simulink model "verify_Flow_Mixer_Thermostatic_mdl"  (R2016b)
settings: Solver=ode45  StartTime=0.0  StopTime=600  MaxStep=1  RelTol=1e-3  EnableMultiTasking=on
libraries: carnot x7, simulink x2
settings Model: DEBUGGLOBALLEVEL=NOLEVEL  DEBUGMAXTOTALWARNINGS=inf  DEBUGMAXCONSECUTIVEWARNINGS=inf  DEBUGWRITETOFILE=0  DEBUGFILENAME='error.txt'  Creator=drhf  LastModifiedBy=drhf
settings DataIOCC: SaveFormat=Array  SignalLoggingSaveFormat=ModelDataLogs
settings OptimizationCC: ExpressionDepthLimit=2147483647  LifeSpan=inf
settings DebuggingCC: UnderspecifiedInitializationDetection=Classic  MergeDetectMultiDrivingBlocksExec=none  SolverPrmCheckMsg=warning  FcnCallInpInsideContextMsg=warning  StateNameClashWarn=warning  SFUnexpectedBacktrackingDiag=warning  SFNoUnconditionalDefaultTransitionDiag=warning  SFExecutionAtInitializationDiag=none
settings HardwareCC: ProdBitPerPointer=32  ProdBitPerSizeT=32  ProdBitPerPtrDiffT=32  ProdLargestAtomicFloat=None  ProdIntDivRoundTo=Undefined  ProdEndianess=Unspecified  ProdWordSize=32  ProdHWDeviceType=32-bit Generic
settings ModelReferenceCC: PropagateSignalLabelsOutOfModel=off
settings GRTTargetCC: TargetLangStandard=C89/C90 (ANSI)  GeneratePreprocessorConditionals=Disable all  CombineOutputUpdateFcns=off  GRTInterface=on
settings ConfigComp: CovMetricSettings=dw  CovHtmlReporting=on  CovSaveCumulativeToWorkspaceVar=on  CovSaveSingleToWorkspaceVar=on  CovExternalEMLEnable=off

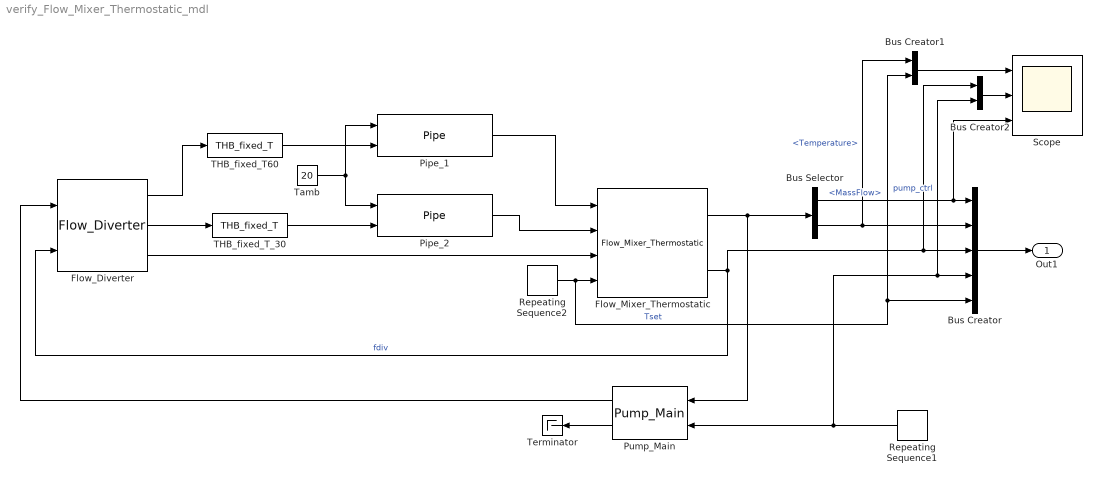
== system verify_Flow_Mixer_Thermostatic_mdl ==
  Bus Creator : BusCreator  Inputs=5
  Bus Creator1 : BusCreator  Inputs=2
  Bus Creator2 : BusCreator  Inputs=2
  Bus Selector : BusSelector  OutputSignals=MassFlow,Temperature
  Flow_Diverter : carnot/Hydraulics/Flow_Diverter
  Flow_Mixer_Thermostatic : carnot/Hydraulics/Flow_Mixer_Thermostatic  t=10
  Pipe_1 : carnot/Hydraulics/Pipe  dia=0.02  len=10  hgt=5  uloss=100/20/10  cond=0  cwall=1000  t0=20  lin=100/0.2  qua=100/0.2^2  nodes=10
  Pipe_2 : carnot/Hydraulics/Pipe  dia=0.02  len=10  hgt=5  uloss=100/20/10  cond=0  cwall=1000  t0=20  lin=100/0.2  qua=100/0.2^2  nodes=10
  Pump_Main : carnot/Hydraulics/Pump_Main  a0=2.7e4  a1=-1.2e4  a2=0%-3e-3  dia=0.025  t1=5  p0=3e5  IDchk=off  fluid_id=Water  mix=0  mix2=0  mix3=0  ua=1  mcp=500  tamb=20
  Repeating Sequence1 : simulink/Sources/Repeating Sequence  rep_seq_t=[ 0 195 195.1 202 202.1 601]  rep_seq_y=[ 1 1 0 0 1 1]
  Repeating Sequence2 : simulink/Sources/Repeating Sequence  rep_seq_t=[0 300 350 601]  rep_seq_y=[50 50 35 35]
  Scope : Scope  NumInputPorts=3
  THB_fixed_T60 : carnot/Source/Simple/THB_fixed_T  t=60
  THB_fixed_T_30 : carnot/Source/Simple/THB_fixed_T  t=30
  Tamb : Constant  Value=20
  Terminator : Terminator
  Out1 : Outport
  wires:
  Bus Creator/1 -> Out1/1
  Flow_Mixer_Thermostatic/1 -> Bus Selector/1, Pump_Main/1
  Bus Selector/1 -> Scope/3, Bus Creator/1  "<MassFlow>"
  Bus Selector/2 -> Bus Creator1/1, Bus Creator/2  "<Temperature>"
  Flow_Mixer_Thermostatic/2 -> Flow_Diverter/2, Bus Creator2/1, Bus Creator/3  "fdiv"
  Tamb/1 -> Pipe_1/1, Pipe_2/1
  Pipe_1/1 -> Flow_Mixer_Thermostatic/1
  THB_fixed_T60/1 -> Pipe_1/2
  THB_fixed_T_30/1 -> Pipe_2/2
  Pipe_2/1 -> Flow_Mixer_Thermostatic/2
  Flow_Diverter/1 -> THB_fixed_T60/1
  Flow_Diverter/2 -> THB_fixed_T_30/1
  Flow_Diverter/3 -> Flow_Mixer_Thermostatic/3
  Repeating Sequence1/1 -> Bus Creator2/2, Bus Creator/4, Pump_Main/2  "pump_ctrl"
  Pump_Main/2 -> Terminator/1
  Pump_Main/1 -> Flow_Diverter/1
  Repeating Sequence2/1 -> Bus Creator/5, Bus Creator1/2, Flow_Mixer_Thermostatic/4  "Tset"
  Bus Creator1/1 -> Scope/1
  Bus Creator2/1 -> Scope/2
